simulink library "fluidDynamicSurfacePool_cl"  (R2020a)
settings: Solver=VariableStepAuto  StartTime=0.0  StopTime=10.0  RelTol=1e-3
undefined symbols (not defined in the file or in its folder): env, vcl
libraries: calcFluidDynamicLoadsPool x2, calcFluidDynamicLoads x2
settings Model: Creator=mcobb  LastModifiedBy=andre
settings DataIOCC: ReturnWorkspaceOutputs=off
settings DebuggingCC: ArithmeticOperatorsInVariantConditions=warning
settings SFSimCC: CustomCodeUndefinedFunction=UseInterfaceOnly

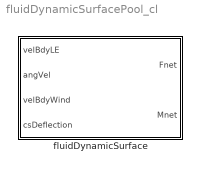
== system fluidDynamicSurfacePool_cl ==
  fluidDynamicSurface : Subsystem  mask{vcl=vcl, fluidDensity=env.water.density.Value, fluidMomentArms=vcl.fluidMomentArms.Value, fluidRefArea=vcl.fluidRefArea.Value, wingTips=vcl.wingTipPositions.Value}
      mask prompts: vcl "Vehicle object"; fluidDensity "Fluid density"; fluidMomentArms "Fluid Moment Arms"; fluidRefArea "Fluid Reference Area"; wingTips "Wing Tips"
      mask help:
      | Input must be an 1×N struct array with fields:
      |     refArea
      |     aeroCentPosVec
      |     spanUnitVec
      |     chordUnitVec
      |     CL
      |     CD
      |     alpha
      |     GainCL
      |     GainCD
      |
      | where N is the number of aerodynamic surfaces
      settings: MinAlgLoopOccurrences=on

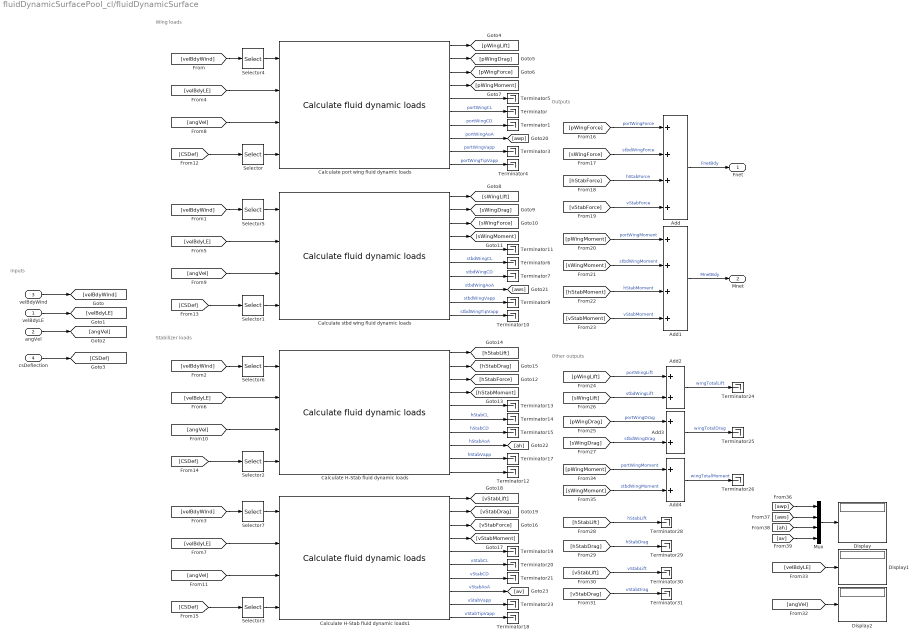
== system fluidDynamicSurfacePool_cl/fluidDynamicSurface ==
  note: Other outputs
  note: Outputs
  note: WIng loads
  note: Stabilizer loads
  note: inputs
  velBdyLE : Inport
  angVel : Inport  Port=2
  velBdyWind : Inport  Port=3
  csDeflection : Inport  Port=4
  Add : Sum  Inputs=++++
  Add1 : Sum  Inputs=++++
  Add2 : Sum
  Add3 : Sum
  Add4 : Sum
  Calculate H-Stab fluid dynamic loads : calcFluidDynamicLoadsPool/Calculate fluid dynamic loads  aSurf=vcl.hStab  sRef=fluidRefArea  rArm_LE=fluidMomentArms(:,3)  rTip_LE=wingTips(:,3)  fluidDensity=fluidDensity
  Calculate H-Stab fluid dynamic loads1 : calcFluidDynamicLoadsPool/Calculate fluid dynamic loads  aSurf=vcl.vStab  sRef=fluidRefArea  rArm_LE=fluidMomentArms(:,4)  rTip_LE=wingTips(:,4)  fluidDensity=fluidDensity
      link override Subsystem: aSurf=aSurf
  Calculate port wing fluid dynamic loads : calcFluidDynamicLoads/Calculate fluid dynamic loads  aSurf=vcl.portWing  sRef=fluidRefArea  rArm_LE=fluidMomentArms(:,1)  rTip_LE=wingTips(:,1)  fluidDensity=fluidDensity
  Calculate stbd wing fluid dynamic loads : calcFluidDynamicLoads/Calculate fluid dynamic loads  aSurf=vcl.stbdWing  sRef=fluidRefArea  rArm_LE=fluidMomentArms(:,2)  rTip_LE=wingTips(:,2)  fluidDensity=fluidDensity
  Display : Display
  Display1 : Display
  Display2 : Display
  Mux : Mux
  Selector : Selector  InputPortWidth=4  IndexOptions=Index vector (dialog)  Indices=1  OutputSizes=1
  Selector1 : Selector  InputPortWidth=4  IndexOptions=Index vector (dialog)  Indices=2  OutputSizes=1
  Selector2 : Selector  InputPortWidth=4  IndexOptions=Index vector (dialog)  Indices=3  OutputSizes=1
  Selector3 : Selector  InputPortWidth=4  IndexOptions=Index vector (dialog)  Indices=4  OutputSizes=1
  Selector4 : Selector  NumberOfDimensions=2  InputPortWidth=4  IndexOptions=Select all,Index vector (dialog)  Indices=1,1  OutputSizes=1,1
  Selector5 : Selector  NumberOfDimensions=2  InputPortWidth=4  IndexOptions=Select all,Index vector (dialog)  Indices=1,2  OutputSizes=1,1
  Selector6 : Selector  NumberOfDimensions=2  InputPortWidth=4  IndexOptions=Select all,Index vector (dialog)  Indices=1,3  OutputSizes=1,1
  Selector7 : Selector  NumberOfDimensions=2  InputPortWidth=4  IndexOptions=Select all,Index vector (dialog)  Indices=1,4  OutputSizes=1,1
  Terminator{,1,3..7,9..15,17..21,23..26,28..31} (27 alike) : Terminator
  Fnet : Outport
  Mnet : Outport  Port=2
  wires:
  angVel/1 -> [angVel]
  velBdyLE/1 -> [velBdyLE]
  velBdyWind/1 -> [velBdyWind]
  csDeflection/1 -> [CSDef]
  [velBdyWind] -> Selector4/1
  [velBdyWind] -> Selector5/1
  [velBdyWind] -> Selector6/1
  [velBdyWind] -> Selector7/1
  [velBdyLE] -> Calculate port wing fluid dynamic loads/2
  [velBdyLE] -> Calculate stbd wing fluid dynamic loads/2
  [velBdyLE] -> Calculate H-Stab fluid dynamic loads/2
  [velBdyLE] -> Calculate H-Stab fluid dynamic loads1/2
  [angVel] -> Calculate port wing fluid dynamic loads/3
  [angVel] -> Calculate stbd wing fluid dynamic loads/3
  [angVel] -> Calculate H-Stab fluid dynamic loads/3
  [angVel] -> Calculate H-Stab fluid dynamic loads1/3
  [CSDef] -> Selector/1
  Selector/1 -> Calculate port wing fluid dynamic loads/4
  Selector1/1 -> Calculate stbd wing fluid dynamic loads/4
  [CSDef] -> Selector1/1
  [CSDef] -> Selector2/1
  [CSDef] -> Selector3/1
  Selector2/1 -> Calculate H-Stab fluid dynamic loads/4
  Selector3/1 -> Calculate H-Stab fluid dynamic loads1/4
  Calculate port wing fluid dynamic loads/1 -> [pWingLift]
  Calculate port wing fluid dynamic loads/2 -> [pWingDrag]
  Calculate port wing fluid dynamic loads/3 -> [pWingForce]
  Calculate port wing fluid dynamic loads/4 -> [pWingMoment]
  Calculate port wing fluid dynamic loads/6 -> Terminator/1  "portWingCL"
  Calculate port wing fluid dynamic loads/7 -> Terminator1/1  "portWingCD"
  Calculate port wing fluid dynamic loads/8 -> [awp]  "portWingAoA"
  Calculate port wing fluid dynamic loads/9 -> Terminator3/1  "portWingVapp"
  Calculate port wing fluid dynamic loads/10 -> Terminator4/1  "portWingTipVapp"
  Calculate port wing fluid dynamic loads/5 -> Terminator5/1
  Calculate stbd wing fluid dynamic loads/5 -> Terminator11/1
  Calculate stbd wing fluid dynamic loads/9 -> Terminator9/1  "stbdWingVapp"
  Calculate stbd wing fluid dynamic loads/6 -> Terminator6/1  "stbdWingCL"
  Calculate stbd wing fluid dynamic loads/8 -> [aws]  "stbdWingAoA"
  Calculate stbd wing fluid dynamic loads/7 -> Terminator7/1  "stbdWingCD"
  Calculate stbd wing fluid dynamic loads/10 -> Terminator10/1  "stbdWingTipVapp"
  Calculate stbd wing fluid dynamic loads/1 -> [sWingLift]
  Calculate stbd wing fluid dynamic loads/2 -> [sWingDrag]
  Calculate stbd wing fluid dynamic loads/3 -> [sWingForce]
  Calculate stbd wing fluid dynamic loads/4 -> [sWingMoment]
  Calculate H-Stab fluid dynamic loads/2 -> [hStabDrag]
  Calculate H-Stab fluid dynamic loads/5 -> Terminator13/1
  Calculate H-Stab fluid dynamic loads/10 -> Terminator12/1
  Calculate H-Stab fluid dynamic loads/1 -> [hStabLift]
  Calculate H-Stab fluid dynamic loads/6 -> Terminator14/1  "hStabCL"
  Calculate H-Stab fluid dynamic loads/3 -> [hStabForce]
  Calculate H-Stab fluid dynamic loads/8 -> [ah]  "hStabAoA"
  Calculate H-Stab fluid dynamic loads/9 -> Terminator17/1  "hStabVapp"
  Calculate H-Stab fluid dynamic loads1/3 -> [vStabForce]
  Calculate H-Stab fluid dynamic loads1/1 -> [vStabLift]
  Calculate H-Stab fluid dynamic loads1/6 -> Terminator20/1  "vStabCL"
  Calculate H-Stab fluid dynamic loads1/9 -> Terminator23/1  "vStabVapp"
  Calculate H-Stab fluid dynamic loads1/4 -> [vStabMoment]
  Calculate H-Stab fluid dynamic loads1/8 -> [av]  "vStabAoA"
  Calculate H-Stab fluid dynamic loads1/5 -> Terminator19/1
  Calculate H-Stab fluid dynamic loads1/2 -> [vStabDrag]
  Calculate H-Stab fluid dynamic loads1/10 -> Terminator18/1  "vStabTipVapp"
  Calculate H-Stab fluid dynamic loads1/7 -> Terminator21/1  "vStabCD"
  [pWingForce] -> Add/1  "portWingForce"
  [sWingForce] -> Add/2  "stbdWingForce"
  [vStabForce] -> Add/4  "vStabForce"
  [hStabForce] -> Add/3  "hStabForce"
  Add/1 -> Fnet/1  "FnetBdy"
  Add1/1 -> Mnet/1  "MnetBdy"
  [vStabMoment] -> Add1/4  "vStabMoment"
  [hStabMoment] -> Add1/3  "hStabMoment"
  [sWingMoment] -> Add1/2  "stbdWingMoment"
  [pWingMoment] -> Add1/1  "portWingMoment"
  [vStabDrag] -> Terminator31/1  "vStabDrag"
  [vStabLift] -> Terminator30/1  "vStabLift"
  [hStabDrag] -> Terminator29/1  "hStabDrag"
  [hStabLift] -> Terminator28/1  "hStabLift"
  [sWingDrag] -> Add3/2  "stbdWingDrag"
  [sWingLift] -> Add2/2  "stbdWingLift"
  [pWingDrag] -> Add3/1  "portWingDrag"
  [pWingLift] -> Add2/1  "portWingLift"
  Selector4/1 -> Calculate port wing fluid dynamic loads/1
  Selector5/1 -> Calculate stbd wing fluid dynamic loads/1
  Selector6/1 -> Calculate H-Stab fluid dynamic loads/1
  Selector7/1 -> Calculate H-Stab fluid dynamic loads1/1
  Add2/1 -> Terminator24/1  "wingTotalLift"
  Add3/1 -> Terminator25/1  "wingTotalDrag"
  Add4/1 -> Terminator26/1  "wingTotalMoment"
  [pWingMoment] -> Add4/1  "portWingMoment"
  [sWingMoment] -> Add4/2  "stbdWingMoment"
  [av] -> Mux/4
  [ah] -> Mux/3
  [aws] -> Mux/2
  [awp] -> Mux/1
  Mux/1 -> Display/1
  [angVel] -> Display2/1
  [velBdyLE] -> Display1/1
  Calculate H-Stab fluid dynamic loads/7 -> Terminator15/1  "hStabCD"
  Calculate H-Stab fluid dynamic loads/4 -> [hStabMoment]
